simulink model "q_sswe_ip02"  (Simulink 7.7)
settings: Solver=ode4  StartTime=0.0  StopTime=inf  FixedStep=0.001  RelTol=1e-3  AbsTol=1e-6
values from neighbouring files (symbols this model uses):
  k = K    (= 15)    [scrap.m]    (also in transfer_functions.m = 1)
undefined symbols (not defined in the file or in its folder): HIL, K_CABLE, K_EC, K_EP, KE_SW, Kgs, MAX_I_WINDUP, MIN_I_WINDUP, parameter_gains, qc_get_step_size, tilt_angle_correction_factor, VMAX_DAC, VMAX_UPM, wcf, X_LIM_ENABLE, X_MAX, X_MIN, zetaf
libraries: quarc_library x6, simulink_extras x4
settings Model: Creator=MLevis  LastModifiedBy=ptwilhelm  SimulationMode=external  ExtModeTrigDuration=10000  ExtModeAutoUpdateStatusClock=off  BufferReuse=off
settings SolverCC: PositivePriorityOrder=on
settings DataIOCC: LimitDataPoints=off
settings OptimizationCC: BooleanDataType=off  InlineInvariantSignals=on  OptimizeBlockIOStorage=off  BufferReuse=off  ExpressionFolding=off  FoldNonRolledExpr=off  LocalBlockOutputs=off  InitFltsAndDblsToZero=on
settings DebuggingCC: SaveWithParameterizedLinksMsg=none  SignalResolutionControl=TryResolveAllWithWarning  SolverPrmCheckMsg=none  MultiTaskDSMMsg=warning  MultiTaskCondExecSysMsg=none  StrictBusMsg=None
settings RTWCC: SystemTargetFile=quarc_win64.tlc  TemplateMakefile=quarc_default_tmf  Description=QUARC Win64 Target  ProcessScript=quarc_win64_make_rtw_hook  IncludeERTFirstTime=on
settings STFCustomTargetCC: TargetPreCompLibLocation=C:\PROGRA~3\QUARC\lib\2011a\win64\release  FunctionExecutionProfile=off  GeneratePreprocessorConditionals=Disable all  SystemTargetFile=quarc_win64.tlc
settings GRTTargetCC: TargetPreCompLibLocation=C:\PROGRA~3\QUARC\lib\2011a\win64\release  ParMdlRefBuildCompliant=off  CompOptLevelCompliant=off  MatFileLogging=off  ExtMode=on  ExtModeMexFile=quarc_comm

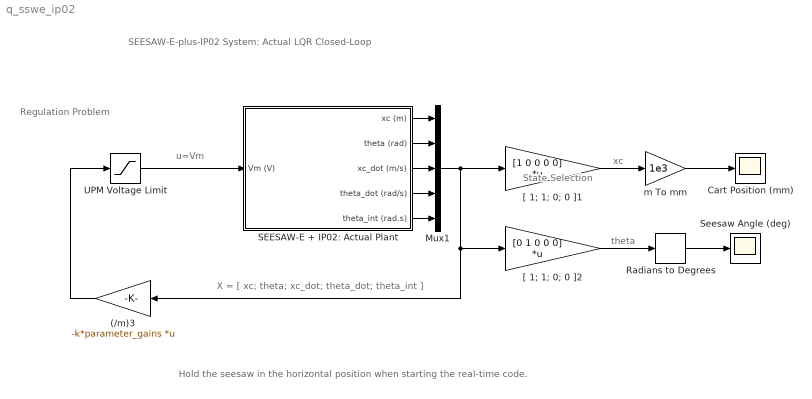
== system q_sswe_ip02 ==
  note: SEESAW-E-plus-IP02 System:
      | Actual LQR Closed-Loop
  note: u=Vm
  note: X = [ xc; theta; xc_dot; theta_dot; theta_int ]
  note: Regulation Problem
  note: xc
  note: State Selection
  note: theta
  note: Hold the seesaw in the horizontal position when starting the real-time code.
  (/m)3 : Gain  Gain=-k*parameter_gains  Multiplication=Matrix(K*u)  SaturateOnIntegerOverflow=on  OutDataTypeStr=Inherit: Same as input  ParamDataTypeStr=Inherit: Same as input
  Cart Position (mm) : Scope
      settings: TickLabels=on  TimeRange=10  YMin=-120  YMax=20  SaveName=data_xc  DataFormat=Array  MaxDataPoints=10000
  Mux1 : Mux  Inputs=5
  Radians to Degrees : simulink_extras/Transformations/Radians to Degrees  SystemSampleTime=-1
  SEESAW-E + IP02: Actual Plant : Subsystem
  Seesaw Angle (deg) : Scope
      settings: TickLabels=on  TimeRange=10  YMin=-4.5  YMax=2  SaveName=data_ssw  DataFormat=Array  MaxDataPoints=10000
  UPM Voltage Limit : Saturate  UpperLimit=VMAX_UPM  LowerLimit=- VMAX_UPM
  "[ 1; 1; 0; 0 ]1" : Gain  Gain=[1 0 0 0 0]  Multiplication=Matrix(K*u)  SaturateOnIntegerOverflow=on  OutDataTypeStr=Inherit: Same as input  ParamDataTypeStr=Inherit: Same as input
  "[ 1; 1; 0; 0 ]2" : Gain  Gain=[0 1 0 0 0]  Multiplication=Matrix(K*u)  SaturateOnIntegerOverflow=on  OutDataTypeStr=Inherit: Same as input  ParamDataTypeStr=Inherit: Same as input
  m To mm : Gain  Gain=1e3  SaturateOnIntegerOverflow=on  OutDataTypeStr=Inherit: Same as input  ParamDataTypeStr=Inherit: Same as input
  wires:
  UPM Voltage Limit/1 -> SEESAW-E + IP02: Actual Plant/1(Vm (V))
  SEESAW-E + IP02: Actual Plant/1(xc (m)) -> Mux1/1
  SEESAW-E + IP02: Actual Plant/4(theta_dot (rad/s)) -> Mux1/4
  Mux1/1 -> "[ 1; 1; 0; 0 ]1"/1, "[ 1; 1; 0; 0 ]2"/1, (/m)3/1
  SEESAW-E + IP02: Actual Plant/3(xc_dot (m/s)) -> Mux1/3
  SEESAW-E + IP02: Actual Plant/2(theta (rad)) -> Mux1/2
  m To mm/1 -> Cart Position (mm)/1
  Radians to Degrees/1 -> Seesaw Angle (deg)/1
  "[ 1; 1; 0; 0 ]2"/1 -> Radians to Degrees/1
  "[ 1; 1; 0; 0 ]1"/1 -> m To mm/1
  (/m)3/1 -> UPM Voltage Limit/1
  SEESAW-E + IP02: Actual Plant/5(theta_int (rad.s)) -> Mux1/5

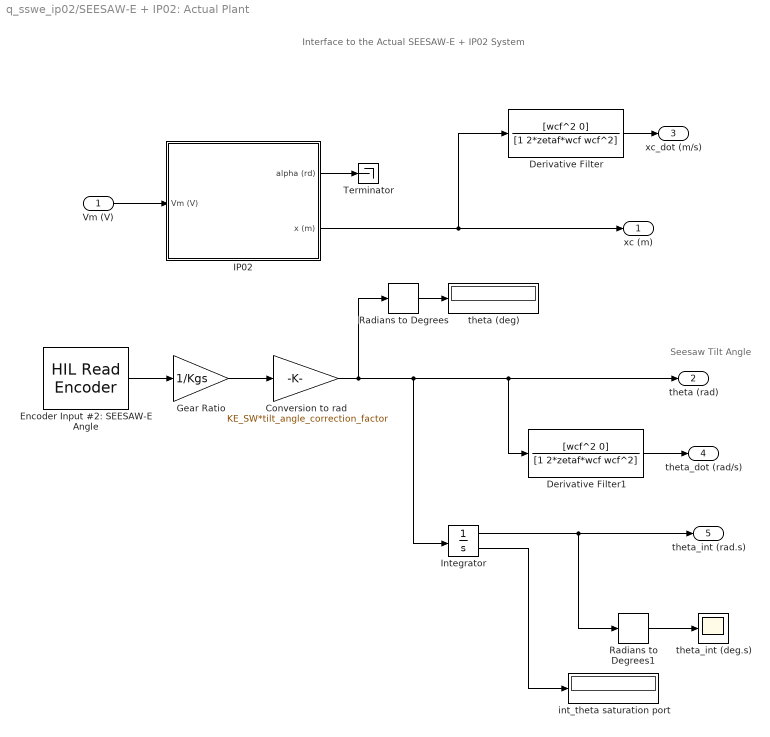
== system q_sswe_ip02/SEESAW-E + IP02: Actual Plant ==
  note: Interface to the Actual
      | SEESAW-E + IP02 System
  note: Seesaw Tilt Angle
  Vm (V) : Inport
  Conversion to rad : Gain  Gain=KE_SW*tilt_angle_correction_factor  SaturateOnIntegerOverflow=on  OutDataTypeStr=Inherit: Same as input  ParamDataTypeStr=Inherit: Same as input
  Derivative Filter : TransferFcn  Numerator=[wcf^2 0]  Denominator=[1 2*zetaf*wcf wcf^2]
  Derivative Filter1 : TransferFcn  Numerator=[wcf^2 0]  Denominator=[1 2*zetaf*wcf wcf^2]
  Encoder Input #2: SEESAW-E Angle : quarc_library/Data Acquisition/Generic/Immediate I//O/HIL Read Encoder  object_name=HIL-1  channels=2  sample_time=qc_get_step_size  active=on  vector_output=off  data_type_mode=Inherit via back propagation  data_type=double
  Gear Ratio : Gain  Gain=1/Kgs  SaturateOnIntegerOverflow=on  OutDataTypeStr=Inherit: Same as input  ParamDataTypeStr=Inherit: Same as input
  "IP02 " : Subsystem
  Integrator : Integrator  LimitOutput=on  UpperSaturationLimit=MAX_I_WINDUP  LowerSaturationLimit=MIN_I_WINDUP  ShowSaturationPort=on
  Radians to Degrees : simulink_extras/Transformations/Radians to Degrees  SystemSampleTime=-1
  Radians to Degrees1 : simulink_extras/Transformations/Radians to Degrees  SystemSampleTime=-1
  Terminator : Terminator
  int_theta saturation port : Display
  theta (deg) : Display
  theta_int (deg.s) : Scope
      settings: TickLabels=on  TimeRange=1.000000  YMin=-250  YMax=250  DataFormat=Array
  xc (m) : Outport  InitialOutput=0
  theta (rad) : Outport  Port=2  InitialOutput=0
  xc_dot (m/s) : Outport  Port=3  InitialOutput=0
  theta_dot (rad/s) : Outport  Port=4  InitialOutput=0
  theta_int (rad.s) : Outport  Port=5  InitialOutput=0
  wires:
  "IP02 "/2(x (m)) -> xc (m)/1, Derivative Filter/1
  Derivative Filter1/1 -> theta_dot (rad/s)/1
  Derivative Filter/1 -> xc_dot (m/s)/1
  Vm (V)/1 -> "IP02 "/1(Vm (V))
  Conversion to rad/1 -> Radians to Degrees/1, theta (rad)/1, Derivative Filter1/1, Integrator/1
  Radians to Degrees/1 -> theta (deg)/1
  Encoder Input #2: SEESAW-E Angle/1 -> Gear Ratio/1
  "IP02 "/1(alpha (rd)) -> Terminator/1
  Gear Ratio/1 -> Conversion to rad/1
  Integrator/1 -> theta_int (rad.s)/1, Radians to Degrees1/1
  Integrator/2 -> int_theta saturation port/1
  Radians to Degrees1/1 -> theta_int (deg.s)/1

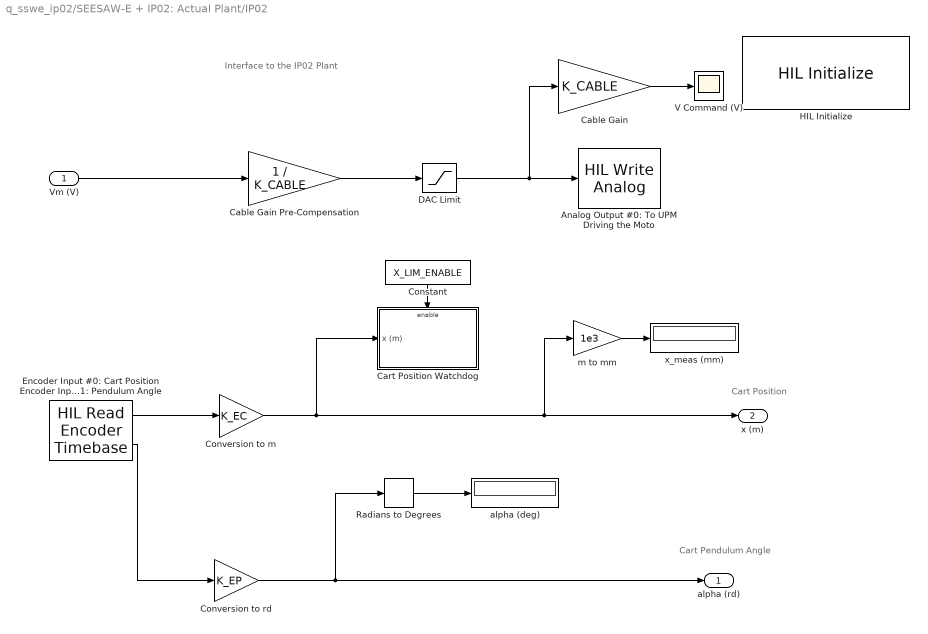
== system q_sswe_ip02/SEESAW-E + IP02: Actual Plant/IP02  ==
  note: Cart Pendulum Angle
  note: Cart Position
  note: Interface to the IP02 Plant
  Vm (V) : Inport
  Analog Output #0: To UPM Driving the Moto : quarc_library/Data Acquisition/Generic/Immediate I//O/HIL Write Analog  Tag=unassigned  object_name=HIL-1  channels=0  sample_time=-1  active=on  vector_input=on
  Cable Gain : Gain  Gain=K_CABLE  SaturateOnIntegerOverflow=on  OutDataTypeStr=Inherit: Same as input  ParamDataTypeStr=Inherit: Same as input
  Cable Gain Pre-Compensation : Gain  Gain=1 / K_CABLE  SaturateOnIntegerOverflow=on  OutDataTypeStr=Inherit: Same as input  ParamDataTypeStr=Inherit: Same as input
  Cart Position Watchdog : Subsystem  TreatAsAtomicUnit=on
  Constant : Constant  Value=X_LIM_ENABLE
  Conversion to m : Gain  Gain=K_EC  SaturateOnIntegerOverflow=on  OutDataTypeStr=Inherit: Same as input  ParamDataTypeStr=Inherit: Same as input
  Conversion to rd : Gain  Gain=K_EP  SaturateOnIntegerOverflow=on  OutDataTypeStr=Inherit: Same as input  ParamDataTypeStr=Inherit: Same as input
  DAC Limit : Saturate  UpperLimit=VMAX_DAC  LowerLimit=- VMAX_DAC
  Encoder Input #0: Cart Position Encoder Input #1: Pendulum Angle : quarc_library/Data Acquisition/Generic/Timebases/HIL Read Encoder Timebase  Tag=unassigned  object_name=HIL-1  clock=0  channels=[0 1]  samples_in_buffer=max(ceil(1/qc_get_step_size), 1)  active=on  vector_output=off  data_type_mode=Inherit via back propagation  data_type=double
  HIL Initialize : quarc_library/Data Acquisition/Generic/Configuration/HIL Initialize  object_name=HIL-1  board_type=q8_usb  board_number=0  board_options=update_rate=normal;decimation=1  exclusive=off  active=on  hardware_clocks=[0:2]  clock_modes=[]  initial_clock_frequencies=[]  set_clock_params_at_start=off  set_clock_params_at_switch_in=off  set_clock_frequencies_at_start=off  set_clock_frequencies_at_switch_in=off  analog_input_channels=[0:7]  analog_input_maximums=10  analog_input_minimums=-10  set_analog_input_params_at_start=on  set_analog_input_params_at_switch_in=off  analog_output_channels=[0:7]  analog_output_maximums=10  analog_output_minimums=-10  initial_analog_outputs=[0]  final_analog_outputs=[0]  watchdog_analog_outputs=0  set_analog_output_params_at_start=on  set_analog_output_params_at_switch_in=off  set_analog_outputs_at_start=on  set_analog_outputs_at_switch_in=off  set_analog_outputs_at_terminate=on  set_analog_outputs_at_switch_out=off  set_analog_outputs_on_watchdog=off  digital_input_channels=[]  digital_output_channels=[]  digital_output_configuration=[]  initial_digital_outputs=[1]  final_digital_outputs=[1]  watchdog_digital_outputs=[1]  set_digital_output_params_at_start=off  set_digital_output_params_at_switch_in=off  set_digital_outputs_at_start=on  set_digital_outputs_at_switch_in=off  set_digital_outputs_at_terminate=on  set_digital_outputs_at_switch_out=off  set_digital_outputs_on_watchdog=off  encoder_channels=[0:7]  quadrature=[4]  encoder_filter_frequency=[]  initial_encoder_counts=[0]  set_encoder_params_at_start=on  set_encoder_params_at_switch_in=off  set_encoder_counts_at_start=on  set_encoder_counts_at_switch_in=off  pwm_channels=[0:7]  pwm_modes=0  pwm_frequency=99.532799999999995e6/4095  pwm_configuration=[0]  pwm_alignment=[0]  pwm_polarity=[1]  pwm_leading_deadband=[0]  pwm_trailing_deadband=[0]  initial_pwm_outputs=[0]  final_pwm_outputs=[0]  watchdog_pwm_outputs=[0]  set_pwm_params_at_start=on  set_pwm_params_at_switch_in=off  set_pwm_outputs_at_start=on  set_pwm_outputs_at_switch_in=off  set_pwm_outputs_at_terminate=on  set_pwm_outputs_at_switch_out=off  set_pwm_outputs_on_watchdog=off  other_output_channels=[]  initial_other_outputs=[]  final_other_outputs=[]  watchdog_other_outputs=[]  set_other_outputs_at_start=off  set_other_outputs_at_switch_in=off  set_other_outputs_at_terminate=off  set_other_outputs_at_switch_out=off  set_other_outputs_on_watchdog=off
  Radians to Degrees : simulink_extras/Transformations/Radians to Degrees  SystemSampleTime=-1
  V Command (V) : Scope
      settings: TickLabels=on  TimeRange=10  SaveName=data_Vm  DataFormat=Array  MaxDataPoints=10000
  alpha (deg) : Display
  m to mm : Gain  Gain=1e3  SaturateOnIntegerOverflow=on  OutDataTypeStr=Inherit: Same as input  ParamDataTypeStr=Inherit: Same as input
  x_meas (mm) : Display
  alpha (rd) : Outport  InitialOutput=0
  x (m) : Outport  Port=2  InitialOutput=0
  wires:
  Encoder Input #0: Cart Position Encoder Input #1: Pendulum Angle/1 -> Conversion to m/1
  Conversion to m/1 -> Cart Position Watchdog/1(x (m)), x (m)/1, m to mm/1
  Cable Gain Pre-Compensation/1 -> DAC Limit/1
  m to mm/1 -> x_meas (mm)/1
  Encoder Input #0: Cart Position Encoder Input #1: Pendulum Angle/2 -> Conversion to rd/1
  Radians to Degrees/1 -> alpha (deg)/1
  Conversion to rd/1 -> Radians to Degrees/1, alpha (rd)/1
  Constant/1 -> Cart Position Watchdog/Enable
  DAC Limit/1 -> Analog Output #0: To UPM Driving the Moto/1, Cable Gain/1
  Vm (V)/1 -> Cable Gain Pre-Compensation/1
  Cable Gain/1 -> V Command (V)/1

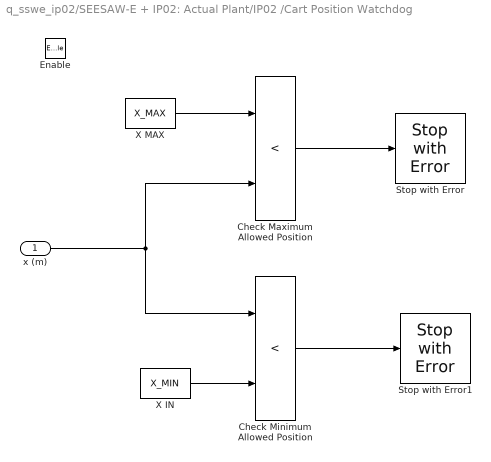
== system q_sswe_ip02/SEESAW-E + IP02: Actual Plant/IP02 /Cart Position Watchdog ==
  x (m) : Inport
  Enable : EnablePort
  Check Maximum Allowed Position : RelationalOperator  Operator=<  InputSameDT=on
  Check Minimum Allowed Position : RelationalOperator  Operator=<  InputSameDT=on
  Stop with Error : quarc_library/Sinks/Error Handling/Stop with Error  message_type=Fixed error message  message=Maximum Limit Reached.
      settings: AttributesFormatString="\"%<message>\""
  Stop with Error1 : quarc_library/Sinks/Error Handling/Stop with Error  message_type=Fixed error message  message=Minimum Limit Reached.
      settings: AttributesFormatString="\"%<message>\""
  X IN : Constant  Value=X_MIN
  X MAX : Constant  Value=X_MAX
  wires:
  Check Maximum Allowed Position/1 -> Stop with Error/1
  x (m)/1 -> Check Minimum Allowed Position/1, Check Maximum Allowed Position/2
  X IN/1 -> Check Minimum Allowed Position/2
  Check Minimum Allowed Position/1 -> Stop with Error1/1
  X MAX/1 -> Check Maximum Allowed Position/1
